simulink model "estimator"  (R2016a)
settings: Solver=FixedStepDiscrete  StartTime=0.0  StopTime=10.0  RelTol=1e-3
libraries: rvs x48
settings Model: Creator=Arthur  LastModifiedBy=arthur
settings DataIOCC: LimitDataPoints=on  SaveFormat=Array
settings DebuggingCC: SolverPrmCheckMsg=warning
settings HardwareCC: ProdBitPerPointer=32  ProdLargestAtomicFloat=None  ProdIntDivRoundTo=Undefined  ProdEndianess=Unspecified  ProdWordSize=32  ProdHWDeviceType=32-bit Generic
settings ModelReferenceCC: PropagateSignalLabelsOutOfModel=off
settings ConfigComp: CovModelRefEnable=Off  CovSFcnEnable=off

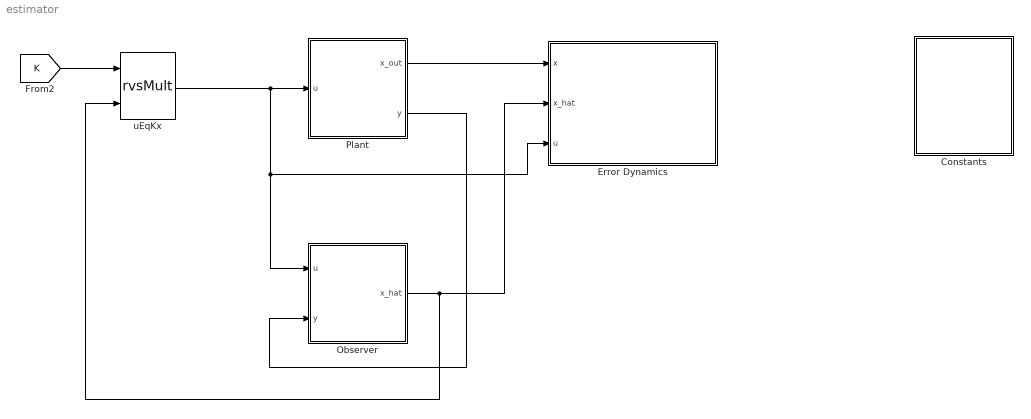
== system estimator ==
  Constants : Subsystem
  Error Dynamics : Subsystem
  Observer : Subsystem
  Plant : Subsystem
  uEqKx : rvs/rvsMult
  wires:
  [K] -> uEqKx/1
  Plant/2(y) -> Observer/2(y)
  Observer/1(x_hat) -> Error Dynamics/2(x_hat), uEqKx/2
  uEqKx/1 -> Error Dynamics/3(u), Observer/1(u), Plant/1(u)
  Plant/1(x_out) -> Error Dynamics/1(x)

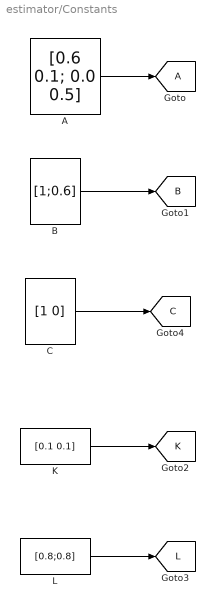
== system estimator/Constants ==
  A : Constant  Value=[0.6 0.1; 0.0 0.5]
  B : Constant  Value=[1;0.6]  VectorParams1D=off
  C : Constant  Value=[1 0]  VectorParams1D=off
  K : Constant  Value=[0.1 0.1]  VectorParams1D=off
  L : Constant  Value=[0.8;0.8]  VectorParams1D=off
  tag scope: A=global, B=global, C=global, K=global, L=global
  wires:
  A/1 -> [A]
  B/1 -> [B]
  K/1 -> [K]
  L/1 -> [L]
  C/1 -> [C]

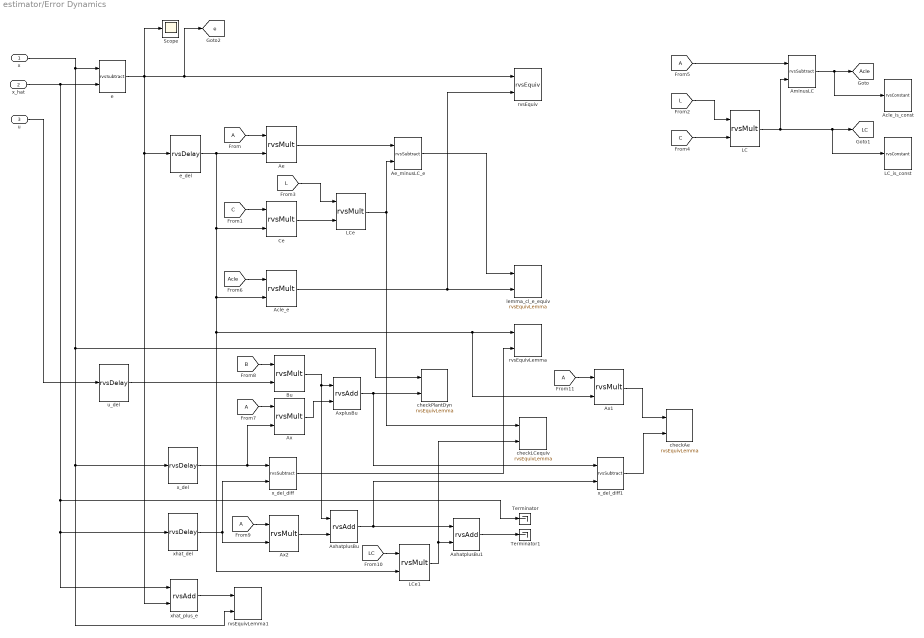
== system estimator/Error Dynamics ==
  x : Inport
  x_hat : Inport  Port=2
  u : Inport  Port=3
  Acle_e : rvs/rvsMult
  Acle_is_const : rvs/rvsConstant
  Ae : rvs/rvsMult
  Ae_minusLC_e : rvs/rvsSubtract
  AminusLC : rvs/rvsSubtract
  Ax : rvs/rvsMult
  Ax1 : rvs/rvsMult
  Ax2 : rvs/rvsMult
  AxhatplusBu : rvs/rvsAdd
  AxhatplusBu1 : rvs/rvsAdd
  AxplusBu : rvs/rvsAdd
  Bu : rvs/rvsMult
  Ce : rvs/rvsMult
  LC : rvs/rvsMult
  LC_is_const : rvs/rvsConstant
  LCe : rvs/rvsMult
  LCe1 : rvs/rvsMult
  Scope : Scope
  Terminator : Terminator
  Terminator1 : Terminator
  checkAe : rvs/rvsEquivLemma  tol=1e-9  nIgnoreSteps=1
  checkLCequiv : rvs/rvsEquivLemma  tol=1e-9  nIgnoreSteps=1
  checkPlantDyn : rvs/rvsEquivLemma  tol=1e-9  nIgnoreSteps=1
  e : rvs/rvsSubtract
  e_del : rvs/rvsDelay  xInit=[0;0]
  lemma_cl_e_equiv : rvs/rvsEquivLemma  tol=1e-9  nIgnoreSteps=1
  rvsEquiv : rvs/rvsEquiv  tol=1e-9  nIgnoreSteps=1
  rvsEquivLemma : rvs/rvsEquivLemma  tol=1e-9  nIgnoreSteps=1
  rvsEquivLemma1 : rvs/rvsEquivLemma  tol=1e-9  nIgnoreSteps=1
  u_del : rvs/rvsDelay  xInit=0
  x_del : rvs/rvsDelay  xInit=[0;0]
  x_del_diff : rvs/rvsSubtract
  x_del_diff1 : rvs/rvsSubtract
  xhat_del : rvs/rvsDelay  xInit=[0;0]
  xhat_plus_e : rvs/rvsAdd
  tag scope: Acle=global, LC=global, e=global
  wires:
  [A] -> Ae/1
  [C] -> Ce/1
  Ae_minusLC_e/1 -> lemma_cl_e_equiv/1
  e/1 -> [e], rvsEquiv/1, Scope/1, xhat_plus_e/2, e_del/1
  LCe/1 -> checkLCequiv/1, Ae_minusLC_e/2
  Ae/1 -> Ae_minusLC_e/1
  e_del/1 -> Acle_e/2, LCe1/2, Ax1/2, rvsEquivLemma/1, Ce/2, Ae/2
  Ce/1 -> LCe/2
  x_hat/1 -> Terminator/1, xhat_plus_e/1, xhat_del/1, e/2
  x/1 -> checkPlantDyn/1, rvsEquivLemma1/2, x_del/1, e/1
  [L] -> LCe/1
  x_del/1 -> x_del_diff/1, Ax/2
  xhat_del/1 -> Ax2/2, x_del_diff/2
  x_del_diff/1 -> rvsEquivLemma/2
  LC/1 -> LC_is_const/1, [LC], AminusLC/2
  [L] -> LC/1
  [C] -> LC/2
  [A] -> AminusLC/1
  AminusLC/1 -> Acle_is_const/1, [Acle]
  [Acle] -> Acle_e/1
  Acle_e/1 -> rvsEquiv/2, lemma_cl_e_equiv/2
  xhat_plus_e/1 -> rvsEquivLemma1/1
  [A] -> Ax/1
  [B] -> Bu/1
  u/1 -> u_del/1
  Bu/1 -> AxhatplusBu/1, AxplusBu/1
  Ax/1 -> AxplusBu/2
  AxplusBu/1 -> x_del_diff1/1, checkPlantDyn/2
  u_del/1 -> Bu/2
  [A] -> Ax2/1
  Ax2/1 -> AxhatplusBu/2
  [LC] -> LCe1/1
  AxhatplusBu/1 -> x_del_diff1/2, AxhatplusBu1/1
  LCe1/1 -> checkLCequiv/2, AxhatplusBu1/2
  AxhatplusBu1/1 -> Terminator1/1
  [A] -> Ax1/1
  Ax1/1 -> checkAe/1
  x_del_diff1/1 -> checkAe/2

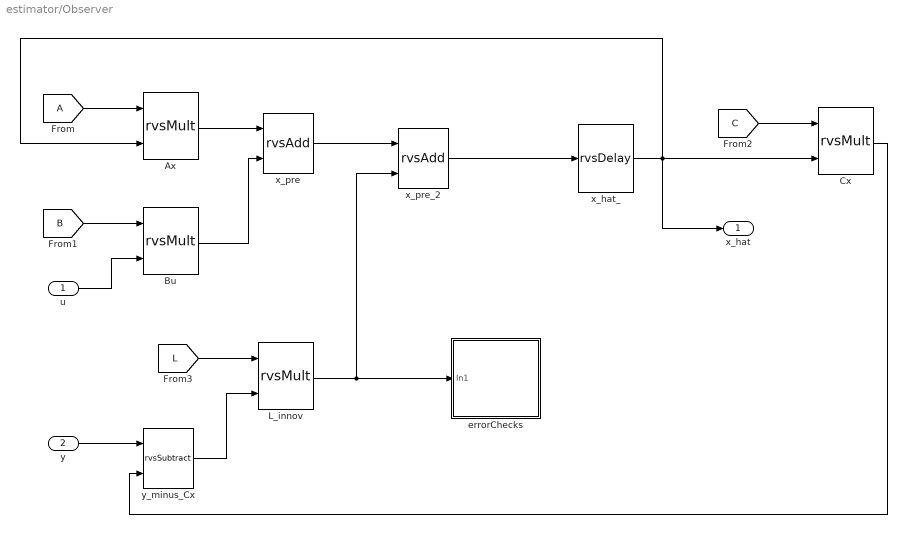
== system estimator/Observer ==
  u : Inport
  y : Inport  Port=2
  Ax : rvs/rvsMult
  Bu : rvs/rvsMult
  Cx : rvs/rvsMult
  L_innov : rvs/rvsMult
  errorChecks : Subsystem
  x_hat_ : rvs/rvsDelay  xInit=[0;0]
  x_pre : rvs/rvsAdd
  x_pre_2 : rvs/rvsAdd
  y_minus_Cx : rvs/rvsSubtract
  x_hat : Outport
  wires:
  Cx/1 -> y_minus_Cx/2
  [C] -> Cx/1
  x_hat_/1 -> Ax/2, x_hat/1, Cx/2
  u/1 -> Bu/2
  Bu/1 -> x_pre/2
  Ax/1 -> x_pre/1
  [A] -> Ax/1
  [B] -> Bu/1
  x_pre/1 -> x_pre_2/1
  x_pre_2/1 -> x_hat_/1
  [L] -> L_innov/1
  y/1 -> y_minus_Cx/1
  y_minus_Cx/1 -> L_innov/2
  L_innov/1 -> x_pre_2/2, errorChecks/1(In1)

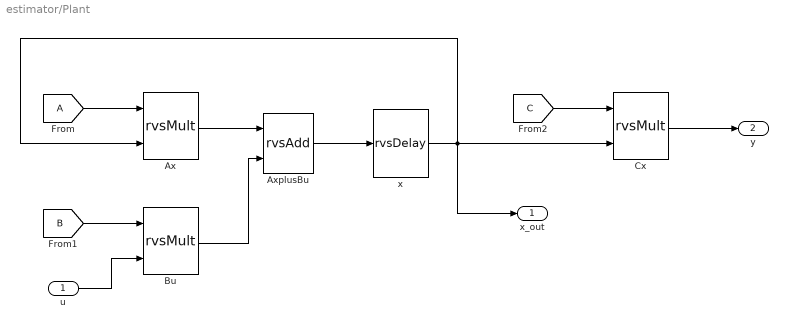
== system estimator/Plant ==
  u : Inport
  Ax : rvs/rvsMult
  AxplusBu : rvs/rvsAdd
  Bu : rvs/rvsMult
  Cx : rvs/rvsMult
  x : rvs/rvsDelay  xInit=[0.7;-1.5]
  x_out : Outport
  y : Outport  Port=2
  wires:
  [B] -> Bu/1
  [A] -> Ax/1
  Ax/1 -> AxplusBu/1
  Bu/1 -> AxplusBu/2
  u/1 -> Bu/2
  AxplusBu/1 -> x/1
  x/1 -> Cx/2, x_out/1, Ax/2
  [C] -> Cx/1
  Cx/1 -> y/1

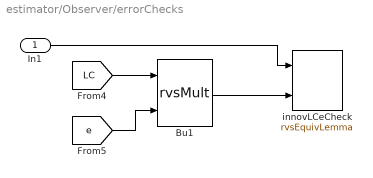
== system estimator/Observer/errorChecks ==
  In1 : Inport
  Bu1 : rvs/rvsMult
  innovLCeCheck : rvs/rvsEquivLemma  tol=1e-9  nIgnoreSteps=1
  wires:
  [e] -> Bu1/2
  In1/1 -> innovLCeCheck/1
  [LC] -> Bu1/1
  Bu1/1 -> innovLCeCheck/2
